simulink model "sm_boom_lift_crawler_harness_ground_manifold_hydr_debug"  (R2024b)
settings: Solver=ode23t  StartTime=0.0  StopTime=tVec.StopTime  FixedStep=2e-3  MaxStep=2  RelTol=1e-3  AbsTol=1e-3
PostLoadFcn:
  | sm_boom_lift_crawler_settest('chassis test')
StartFcn:
  | tic;
StopFcn:
  | Elapsed_Sim_Time = toc;
  | %disp(['Elapsed Sim Time = ' num2str(Elapsed_Sim_Time)]);
undefined symbols (not defined in the file): BasketR, Boom, Chassis, Extend, Jib, LevelM, LevelS, Lift, OutFL, OutFR, OutRL, OutRR, oVec, Tilt, TrackL, TrackR, Turret, tVec
libraries: sm_boom_lift_crawler_lib x22, fl_lib x15, sh_lib x15, nesl_utility x5, sm_lib x2, sm_boom_lift_crawler_lib_lift x1, sm_boom_lift_crawler_lib_inputs x1
(part 1 of 2)
Description:
  | Boom Lift Crawler Chassis with Hydraulic Actuation (Test Harness)
  | 
  | Copyright 2020-2024 The MathWorks, Inc.
settings Model: LastModifiedBy=smiller
settings SolverCC: AutoScaleAbsTol=off  AlgebraicLoopSolver=TrustRegion
settings DataIOCC: SignalLoggingName=logsout_sm_boom_lift_crawler
settings OptimizationCC: ReuseModelBlockBuffer=off
settings DebuggingCC: UnconnectedInputMsg=warning  UnconnectedOutputMsg=warning  UnconnectedLineMsg=warning
settings ModelReferenceCC: EnableRefExpFcnMdlSchedulingChecks=on
settings RTWCC: GPUComputeCapability=3.5  DLArmComputeVersion=19.05
settings SimscapeCC: SimscapeNominalValues="[{\"value\":\"1\",\"unit\":\"A\"},{\"value\":\"nomval_psi\",\"unit\":\"psi\"},{\"value\":\"1\",\"unit\":\"cm^2\"},{\"value\":\"nomval_cmv3_s\",\"unit\":\"cm^3/s\"},{\"value\":\"1\",\"unit\":\"kJ/kg\"},{\"value\":\"1\",\"unit\":\"kW\"},{\"value\":\"1\",\"unit\":\"l\"},{\"value\":\"nomval_N\",\"unit\":\"N\"},{\"value\":\"nomval_Nm\",\"unit\":\"N*m\"},{\"value\":\"1\",\"unit\":\"V\"}]"  SimscapeLogType=all  SimscapeLogName=simlog_sm_boom_lift_crawler  SimscapeLogLimitData=off  SimscapeOperatingPoint=op_hold4Sec_hydr
settings DiagnosticsConfigSet: SimMechanicsConflictingReferenceFrames=none  SimMechanicsRigidlyBoundBlock=none
settings ExplorerConfigSet: InternalSimMechanicsExplorerSettings="<ExplorerConfiguration><canonicalview>default</canonicalview><AnimationSetting><BasePlaybackSpeed>1.0</BasePlaybackSpeed><PlaybackSpeedFactor>8.0</PlaybackSpeedFactor></AnimationSetting><TilePanel><TileInfo><Tiles Columns=\"1\" Count=\"1\" Rows=\"1\"><Column Weight=\"1\"/><Row Weight=\"1\"/><Tile Height=\"1\" Width=\"1\" X=\"0\" Y=\"0\"/></Tiles></TileInfo><SceneInfo><SceneViewer><BGColor><R>1</R><G>1</G><B>1</B></BGColor><Camera><DoPerspective>on</DoPerspective><Position><X>-12.2424581714389937</X><Y>-0.143345264209557399</Y><Z>4.1505972342390427</Z></Position><Center><X>-4.62122899968606404</X><Y>-0.143345264209557399</Y><Z>4.15059723423904359</Z></Center><Up><X>0</X><Y>0</Y><Z>1</Z></Up><ViewLimDist>1</ViewLimDist><YLim>0.466307658154998583</YLim><XLim>0.828991392275552963</XLim></Camera></SceneViewer></SceneInfo></TilePanel><MechEditorPanel><Cameras><Camera><Id>Camera8</Id><Value><Name>Extend_Knuckle</Name><NativeCamera><PositionTrackingFeature>Lift.Boom.Arms.Telescope.Extend_Cylinder.Transform_Camera_Extend_Knuckle.F</PositionTrackingFeature><CenterTrackingFeature>Lift.Boom.Arms.Telescope.Extend_Cylinder.Transform_Camera_Extend_Knuckle.F</CenterTrackingFeature><UpVectorTrackingFeature>Lift.Boom.Arms.Telescope.Extend_Cylinder.Transform_Camera_Extend_Knuckle.F</UpVectorTrackingFeature><CenterTrackingOrigin>off</CenterTrackingOrigin><CenterTrackingDirection>-X</CenterTrackingDirection><UpVectorTrackingDirection>-Y</UpVectorTrackingDirection></NativeCamera></Value></Camera><Camera><Id>Camera9</Id><Value><Name>Extend_Basket</Name><NativeCamera><PositionTrackingFeature>Lift.Boom.Arms.Telescope.Extend_Cylinder.Transform_Camera_Extend_Basket.F</PositionTrackingFeature><CenterTrackingFeature>Lift.Boom.Arms.Telescope.Extend_Cylinder.Transform_Camera_Extend_Basket.F</CenterTrackingFeature><UpVectorTrackingFeature>Lift.Boom.Arms.Telescope.Extend_Cylinder.Transform_Camera_Extend_Basket.F</UpVectorTrackingFeature><CenterTrackingOrigin>off</CenterTrackingOrigin><CenterTrackingDirection>+X</CenterTrackingDirection><UpVectorTrackingDirection>+Y</UpVectorTrackingDirection></NativeCamera></Value></Camera><Camera><Id>Camera10</Id><Value><Name>Basket_Rotate</Name><NativeCamera><PositionTrackingFeature>Lift.Boom.Basket.Basket_Rotate.Bracket.Reference_Camera_Basket_Rotate_L.R</PositionTrackingFeature><CenterTrackingFeature>Lift.Boom.Basket.Basket_Rotate.Bracket.Reference_Camera_Basket_Rotate_L.R</CenterTrackingFeature><UpVectorTrackingFeature>Mech_Config.World.W</UpVectorTrackingFeature><CenterTrackingOrigin>off</CenterTrackingOrigin><CenterTrackingDirection>-X</CenterTrackingDirection><UpVectorTrackingDirection>+Z</UpVectorTrackingDirection></NativeCamera></Value></Camera><Camera><Id>Camera11</Id><Value><Name>Tilt_Knuckle</Name><NativeCamera><PositionTrackingFeature>Lift.Boom.Arms.Tower.Upper_Knuckle.Reference_Knuckle_Cam.R</PositionTrackingFeature><CenterTrackingFeature>Lift.Boom.Arms.Tower.Upper_Knuckle.Reference_Knuckle_Cam.R</CenterTrackingFeature><UpVectorTrackingFeature>Mech_Config.World.W</UpVectorTrackingFeature><CenterTrackingOrigin>off</CenterTrackingOrigin><CenterTrackingDirection>+Z</CenterTrackingDirection><UpVectorTrackingDirection>+Z</UpVectorTrackingDirection></NativeCamera></Value></Camera><Camera><Id>Camera12</Id><Value><Name>Full Test</Name><NativeCamera><PositionKeyframeSet><Keyframe><Time>0</Time><Value><X>-12.242458171438994</X><Y>-0.1433452642095574</Y><Z>4.1505972342390427</Z></Value></Keyframe><Keyframe><Time>69.026826430124729</Time><Value><X>-14.974593328379619</X><Y>0.0056652615564253064</Y><Z>5.3389029552684786</Z></Value></Keyframe><Keyframe><Time>110.29539843687829</Time><Value><X>-21.00761369699504</X><Y>-0.0057417156870510078</Y><Z>8.0689402037867488</Z></Value></Keyframe><Keyframe><Time>140.70430157635164</Time><Value><X>-31.272784439198116</X><Y>-2.5583130214499052e-10</Y><Z>12.723321478963756</Z></Value></Keyframe><Keyframe><Time>181.77628976806102</Time><Value><X>-31.272784439198116</X><Y>-2.5583130214499052e-10</Y><Z>12.723321478963756</Z></Value></Keyframe><Keyframe><Time>208.0087867386398</Time><Value><X>-23.351505250921551</X><Y>-2.5583182919801497e-10</Y><Z>9.1371534281977738</Z></Value></Keyframe><Keyframe><Time>243.06358572448306</Time><Value><X>-16.577121762622586</X><Y>-2.5583144573665537e-10</Y><Z>6.0702143126734844</Z></Value></Keyframe><Keyframe><Time>273.3415757110605</Time><Value><X>-16.577121762622586</X><Y>-2.5583144573665537e-10</Y><Z>6.0702143126734844</Z></Value></Keyframe><Keyframe><Time>321.2447002217541</Time><Value><X>-13.690590902490033</X><Y>0.01787769923724114</Y><Z>4.7891626503614262</Z></Value></Keyframe><Keyframe><Time>350</Time><Value><X>-13.690590902490033</X><Y>0.01787769923724114</Y><Z>4.7891626503614262</Z></Value></Keyframe></PositionKeyframeSet><CenterKeyframeSet><Keyframe><Time>0</Time><Value><X>-4.621228999686064</X><Y>-0.1433452642095574</Y><Z>4.1505972342390436</Z></Value></Keyframe><Keyframe><Time>69.026826430124729</Time><Value><X>-0.17395018713353672</X><Y>0.0056652615564253064</Y><Z>5.3389029552684786</Z></Value></Keyframe><Keyframe><Time>110.29539843687829</Time><Value><X>-9.0038066291239502</X><Y>-0.0057417156870549491</Y><Z>8.0689402037867524</Z></Value></Keyframe><Keyframe><Time>140.70430157635164</Time><Value><X>-14.136391845814327</X><Y>-2.5583979379462107e-10</Y><Z>12.72332147896376</Z></Value></Keyframe><Keyframe><Time>181.77628976806102</Time><Value><X>-2.3429975002054775</X><Y>-2.5584563781180217e-10</Y><Z>12.723321478963761</Z></Value></Keyframe><Keyframe><Time>208.0087867386398</Time><Value><X>-10.17575261115104</X><Y>-2.5583801743778167e-10</Y><Z>9.1371534281977755</Z></Value></Keyframe><Keyframe><Time>243.06358572448306</Time><Value><X>-0.54476849060194255</X><Y>-2.5583897563257738e-10</Y><Z>6.0702143126734844</Z></Value></Keyframe><Keyframe><Time>273.3415757110605</Time><Value><X>-0.11057247639663359</X><Y>-2.5583917956089291e-10</Y><Z>6.0702143126734844</Z></Value></Keyframe><Keyframe><Time>321.2447002217541</Time><Value><X>-5.3452949964231387</X><Y>0.017877699237237366</Y><Z>4.7891626503614253</Z></Value></Keyframe><Keyframe><Time>350</Time><Value><X>-5.3452949964231387</X><Y>0.017877699237237366</Y><Z>4.7891626503614253</Z></Value></Keyframe></CenterKeyframeSet><UpVectorKeyframeSet><Keyframe><Time>0</Time><Value><X>0</X><Y>0</Y><Z>1</Z></Value></Keyframe><Keyframe><Time>69.026826430124729</Time><Value><X>0</X><Y>0</Y><Z>1</Z></Value></Keyframe><Keyframe><Time>110.29539843687829</Time><Value><X>0</X><Y>0</Y><Z>1</Z></Value></Keyframe><Keyframe><Time>140.70430157635164</Time><Value><X>0</X><Y>0</Y><Z>1</Z></Value></Keyframe><Keyframe><Time>181.77628976806102</Time><Value><X>-2.0731981129868445e-16</X><Y>1.0273382740432149e-31</Y><Z>1</Z></Value></Keyframe><Keyframe><Time>208.0087867386398</Time><Value><X>1.4663775813922931e-57</X><Y>2.9591920320379324e-42</Y><Z>1</Z></Value></Keyframe><Keyframe><Time>243.06358572448306</Time><Value><X>1.3898401336634517e-57</X><Y>2.9591920320379324e-42</Y><Z>1</Z></Value></Keyframe><Keyframe><Time>273.3415757110605</Time><Value><X>1.3898401336605064e-57</X><Y>2.9591920320379324e-42</Y><Z>1</Z></Value></Keyframe><Keyframe><Time>321.2447002217541</Time><Value><X>1.3198478700492623e-57</X><Y>2.9591920320379324e-42</Y><Z>1</Z></Value></Keyframe><Keyframe><Time>350</Time><Value><X>1.0642863113510858e-16</X><Y>-4.813997747953607e-32</Y><Z>1</Z></Value></Keyframe></UpVectorKeyframeSet></NativeCamera></Value></Camera><Camera><Id>Camera13</Id><Value><Name>View_Basket_World</Name><NativeCamera><PositionTrackingFeature>Lift.Boom.Basket.Basket.Reference_Basket_Cam.R</PositionTrackingFeature><CenterTrackingFeature>Mech_Config.World.W</CenterTrackingFeature><UpVectorTrackingFeature>Lift.Boom.Basket.Basket.Reference_Basket_Cam.R</UpVectorTrackingFeature><CenterTrackingOrigin>on</CenterTrackingOrigin><UpVectorTrackingDirection>+Y</UpVectorTrackingDirection></NativeCamera></Value></Camera><Camera><Id>Camera14</Id><Value><Name>View_Worm_Drive</Name><NativeCamera><PositionTrackingFeature>Lift.Boom.Turret.Case.Reference_Worm_Cam.R</PositionTrackingFeature><CenterTrackingFeature>Lift.Boom.Turret.Case.Transform_Worm_Cam.B</CenterTrackingFeature><UpVectorTrackingFeature>Mech_Config.World.W</UpVectorTrackingFeature><CenterTrackingOrigin>on</CenterTrackingOrigin><UpVectorTrackingDirection>+Z</UpVectorTrackingDirection></NativeCamera></Value></Camera><Camera><Id>Camera15</Id><Value><Name>Extend_Retract_Pulley</Name><NativeCamera><PositionTrackingFeature>Lift.Boom.Arms.Telescope.Extend_Cylinder.Reference_Camera_Retract_Pulley.R</PositionTrackingFeature><CenterTrackingFeature>Lift.Boom.Arms.Telescope.Extend_Cylinder.Reference_Camera_Retract_Pulley.R</CenterTrackingFeature><UpVectorTrackingFeature>Lift.Boom.Arms.Telescope.Extend_Cylinder.Reference_Camera_Retract_Pulley.R</UpVectorTrackingFeature><CenterTrackingOrigin>off</CenterTrackingOrigin><CenterTrackingDirection>+Y</CenterTrackingDirection><UpVectorTrackingDirection>+Z</UpVectorTrackingDirection></NativeCamera></Value></Camera><Camera><Id>Camera16</Id><Value><Name>Extend_Extend_Pulley</Name><NativeCamera><PositionTrackingFeature>Lift.Boom.Arms.Telescope.Extend_Cylinder.Reference_Camera_Extend_Pulley.R</PositionTrackingFeature><CenterTrackingFeature>Lift.Boom.Arms.Telescope.Extend_Cylinder.Reference_Camera_Extend_Pulley.R</CenterTrackingFeature><UpVectorTrackingFeature>Lift.Boom.Arms.Telescope.Extend_Cylinder.Reference_Camera_Extend_Pulley.R</UpVectorTrackingFeature><CenterTrackingOrigin>off</CenterTrackingOrigin><CenterTrackingDirection>+Z</CenterTrackingDirection><UpVectorTrackingDirection>-Y</UpVectorTrackingDirection></NativeCamera></Value></Camera><Camera><Id>Camera17</Id><Value><Name>Jib</Name><NativeCamera><PositionTrackingFeature>Lift.Boom.Basket.Jib.Jib_Mount.Reference_Camera_Basket_Jib.R</PositionTrackingFeature><CenterTrackingFeature>Lift.Boom.Basket.Jib.Jib_Mount.Reference_Camera_Basket_Jib.R</CenterTrackingFeature><UpVectorTrackingFeature>Mech_Config.World.W</UpVectorTrackingFeature><CenterTrackingOrigin>off</CenterTrackingOrigin><CenterTrackingDirection>-X</CenterTrackingDirection><UpVectorTrackingDirection>+Z</UpVectorTrackingDirection></NativeCamera></Value></Camera></Cameras><GfxPanelCameraMap><MapElement CameraMLId=\"Camera12\" GfxPanelIndex=\"0\"/></GfxPanelCameraMap><VideoCreator><PlaybackSpeedRatio>8</PlaybackSpeedRatio><FrameRate>30</FrameRate><VideoFormat>MPEG-4</VideoFormat><FrameSize>auto</FrameSize></VideoCreator></MechEditorPanel></ExplorerConfiguration>"

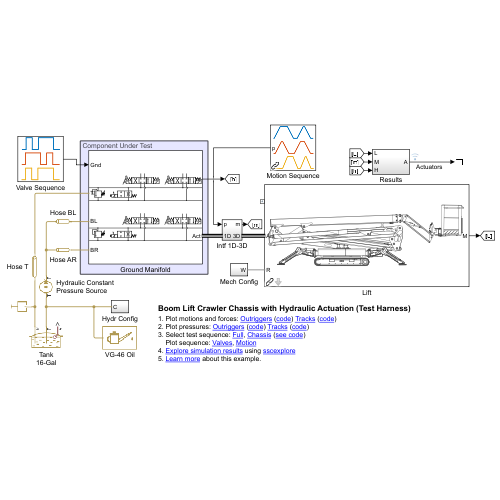
[thumbnail: Simulink's stored preview of the top-level diagram]
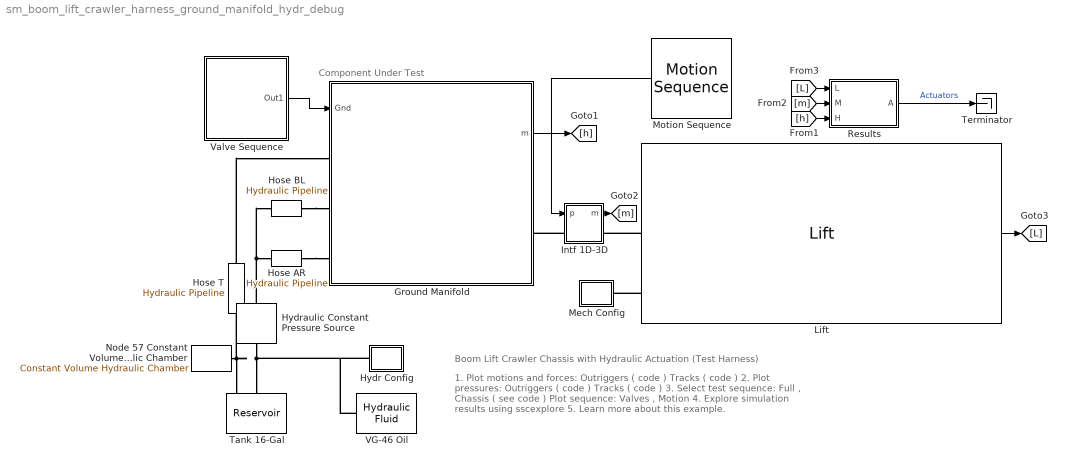
== system sm_boom_lift_crawler_harness_ground_manifold_hydr_debug ==
  note: Component Under Test
  note: Boom Lift Crawler Chassis with Hydraulic Actuation (Test Harness)
  note: 1. Plot motions and forces: Outriggers ( code ) Tracks ( code )
      | 2. Plot pressures: Outriggers ( code ) Tracks ( code )
      | 3. Select test sequence: Full , Chassis ( see code )
      | Plot sequence: Valves , Motion
      | 4. Explore simulation results using sscexplore
      | 5. Learn more about this example.
  Ground Manifold : Subsystem
      mask Display: image('sh004.svg')
  Hose AR : sh_lib/Pipelines/Hydraulic Pipeline  cs_type=1  d_in=lines.ground.main.d.p in  area=1e-4 m^2  D_h=1.12e-2 m  s_factor=64  length=lines.ground.main.l ft  length_ad=lines.ground.main.lr ft  roughness=15e-6 m  Re_lam=2000  Re_turb=4000  wall_type=1  pr_r_coef=2e-12 m/Pa  time_const=0.01 s  k_sh=1.4  initial_pressure=lines.ground.main.p0 psi
      settings: InternalSimscapePortConfiguration="{\"Bottom\":[],\"Left\":[{\"id\":\"A\",\"label\":\"A\",\"type\":\"foundation.hydraulic.hydraulic\"}],\"Right\":[{\"id\":\"B\",\"label\":\"B\",\"type\":\"foundation.hydraulic.hydraulic\"}],\"Top\":[]}"
  Hose BL : sh_lib/Pipelines/Hydraulic Pipeline  cs_type=1  d_in=lines.ground.main.d.p in  area=1e-4 m^2  D_h=1.12e-2 m  s_factor=64  length=lines.ground.main.l ft  length_ad=lines.ground.main.lr ft  roughness=15e-6 m  Re_lam=2000  Re_turb=4000  wall_type=1  pr_r_coef=2e-12 m/Pa  time_const=0.01 s  k_sh=1.4  initial_pressure=lines.ground.main.p0 psi
      settings: InternalSimscapePortConfiguration="{\"Bottom\":[],\"Left\":[{\"id\":\"A\",\"label\":\"A\",\"type\":\"foundation.hydraulic.hydraulic\"}],\"Right\":[{\"id\":\"B\",\"label\":\"B\",\"type\":\"foundation.hydraulic.hydraulic\"}],\"Top\":[]}"
  Hose T : sh_lib/Pipelines/Hydraulic Pipeline  cs_type=1  d_in=lines.ground.main.d.t in  area=1e-4 m^2  D_h=1.12e-2 m  s_factor=64  length=lines.ground.main.l ft  length_ad=lines.ground.main.lr ft  roughness=15e-6 m  Re_lam=2000  Re_turb=4000  wall_type=1  pr_r_coef=2e-12 m/Pa  time_const=0.01 s  k_sh=1.4  initial_pressure=lines.ground.main.p0 psi
      settings: InternalSimscapePortConfiguration="{\"Bottom\":[],\"Left\":[{\"id\":\"A\",\"label\":\"A\",\"type\":\"foundation.hydraulic.hydraulic\"}],\"Right\":[{\"id\":\"B\",\"label\":\"B\",\"type\":\"foundation.hydraulic.hydraulic\"}],\"Top\":[]}"
  Hydr Config : Subsystem
  Hydraulic Constant Pressure Source : fl_lib/Hydraulic/Hydraulic Sources/Hydraulic Constant Pressure Source  commanded_pressure=2e7 Pa
      settings: InternalSimscapePortConfiguration="{\"Bottom\":[],\"Left\":[{\"id\":\"P\",\"label\":\"P\",\"type\":\"foundation.hydraulic.hydraulic\"}],\"Right\":[{\"id\":\"T\",\"label\":\"T\",\"type\":\"foundation.hydraulic.hydraulic\"}],\"Top\":[]}"
  Intf 1D-3D : Subsystem
  Lift : sm_boom_lift_crawler_lib_lift/Lift  popup_gnd_outr=Force
  Mech Config : Subsystem
  Motion Sequence : sm_boom_lift_crawler_lib_inputs/Motion Sequence  SystemSampleTime=-1  VariantActivationTime=update diagram  AllowFlexibleInterface=on  Latency=0  AutoFrameSizeCalculation=off
  Node 57 Constant Volume Hydraulic Chamber : fl_lib/Hydraulic/Hydraulic Elements/Constant Volume Hydraulic Chamber  ch_sp=1  wall_type=1  ch_volume=1e-4 m^3  d_in=1e-2 m  length=1 m  pr_r_coef=1.2e-12 m/Pa  time_const=0.01 s  k_sh=1.4  pressure_specify=off  pressure_priority=High  pressure=0 Pa  pressure_nominal_specify=off  pressure_nominal_value=1  pressure_nominal_unit=Pa  diameter_incr_specify=off  diameter_incr_priority=High  diameter_incr=0 m  diameter_incr_nominal_specify=off  diameter_incr_nominal_value=1  diameter_incr_nominal_unit=m  flow_rate_specify=off  flow_rate_priority=None  flow_rate=0.001 m^3/s  flow_rate_nominal_specify=off  flow_rate_nominal_value=1  flow_rate_nominal_unit=m^3/s
      settings: InternalSimscapePortConfiguration="{\"Bottom\":[],\"Left\":[{\"id\":\"A\",\"label\":\"\",\"type\":\"foundation.hydraulic.hydraulic\"}],\"Right\":[],\"Top\":[]}"
  Results : Subsystem
  "Tank 16-Gal " : sh_lib/Hydraulic Utilities/Reservoir  press=0 psi  init_volume=16 gal  ret_diam=lines.ground.main.d.t in  loss_coeff=1
      settings: InternalSimscapePortConfiguration="{\"Bottom\":[],\"Left\":[{\"id\":\"V\",\"label\":\"V\",\"type\":\"output\"},{\"id\":\"P\",\"label\":\"P\",\"type\":\"foundation.hydraulic.hydraulic\"},{\"id\":\"R\",\"label\":\"R\",\"type\":\"foundation.hydraulic.hydraulic\"}],\"Right\":[],\"Top\":[]}"
  Terminator : Terminator
  VG-46 Oil : sh_lib/Hydraulic Utilities/Hydraulic Fluid  SelFluid=16  SysTemp=40  TrapAir=ratio_dissolved_air  ViscDerFactor=1  range_error=2
  Valve Sequence : Subsystem
      mask Display: image('sm_boom_lift_crawler_valve_seq_outputonly.svg');
  wires:
  Ground Manifold/1(m) -> [h]
  Results/1(A) -> Terminator/1  "Actuators"
  Lift/1 -> [L]
  Valve Sequence/1(Out1) -> Ground Manifold/1(Gnd)
  Motion Sequence/1 -> Intf 1D-3D/1(p)
  [h] -> Results/3(H)
  Intf 1D-3D/1(m) -> [m]
  [m] -> Results/2(M)
  [L] -> Results/1(L)
  connections:
  Hydraulic Constant Pressure Source/RConn1 -- "Tank 16-Gal "/LConn2 -- VG-46 Oil/RConn1 -- Hydr Config/RConn1
  Hose BL/RConn1 -- Ground Manifold/LConn2
  Intf 1D-3D/LConn1 -- Ground Manifold/RConn1
  Hose T/LConn1 -- Ground Manifold/LConn1
  Node 57 Constant Volume Hydraulic Chamber/LConn1 -- "Tank 16-Gal "/LConn3 -- Hose T/RConn1
  Hose AR/RConn1 -- Ground Manifold/LConn3
  Hydraulic Constant Pressure Source/LConn1 -- Hose AR/LConn1 -- Hose BL/LConn1
  Lift/LConn2 -- Intf 1D-3D/RConn1
  Lift/LConn3 -- Mech Config/LConn1

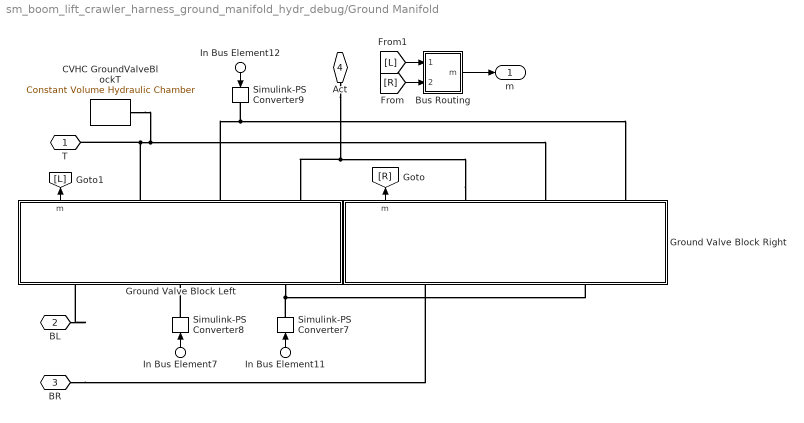
== system sm_boom_lift_crawler_harness_ground_manifold_hydr_debug/Ground Manifold ==
  In Bus Element7 : Inport  PortName=Gnd  Element=Tr
  In Bus Element11 : Inport  PortName=Gnd  Element=Ou
  In Bus Element12 : Inport  PortName=Gnd  Element=Pr
  Bus Routing : Subsystem
  CVHC GroundValveBlockT : fl_lib/Hydraulic/Hydraulic Elements/Constant Volume Hydraulic Chamber  ch_sp=1  wall_type=1  ch_volume=1e-4 m^3  d_in=1e-2 m  length=1 m  pr_r_coef=1.2e-12 m/Pa  time_const=0.01 s  k_sh=1.4  pressure_specify=off  pressure_priority=High  pressure=0 Pa  pressure_nominal_specify=off  pressure_nominal_value=1  pressure_nominal_unit=Pa  diameter_incr_specify=off  diameter_incr_priority=High  diameter_incr=0 m  diameter_incr_nominal_specify=off  diameter_incr_nominal_value=1  diameter_incr_nominal_unit=m  flow_rate_specify=off  flow_rate_priority=None  flow_rate=0.001 m^3/s  flow_rate_nominal_specify=off  flow_rate_nominal_value=1  flow_rate_nominal_unit=m^3/s
      settings: InternalSimscapePortConfiguration="{\"Bottom\":[],\"Left\":[{\"id\":\"A\",\"label\":\"\",\"type\":\"foundation.hydraulic.hydraulic\"}],\"Right\":[],\"Top\":[]}"
  Ground Valve Block Left : Subsystem
      mask Display: image('sh008.svg')
  Ground Valve Block Right : Subsystem
      mask Display: image('sh006.svg')
  Simulink-PS Converter7 : nesl_utility/Simulink-PS Converter  PhysicalDomain=network_engine_domain  SubClassName=ps_input  LeftPortType=input  RightPortType=output  PseudoPeriodic=off  Frequencies=[]  NoiseDistribution=none  NoiseParameters=[]  Unit=1  AffineConversion=off  FilteringAndDerivatives=provide  SimscapeFilterOrder=1  InputFilterTimeConstant=1  UdotUserProvided=0
  Simulink-PS Converter8 : nesl_utility/Simulink-PS Converter  PhysicalDomain=network_engine_domain  SubClassName=ps_input  LeftPortType=input  RightPortType=output  PseudoPeriodic=off  Frequencies=[]  NoiseDistribution=none  NoiseParameters=[]  Unit=1  AffineConversion=off  FilteringAndDerivatives=provide  SimscapeFilterOrder=1  InputFilterTimeConstant=1  UdotUserProvided=0
  Simulink-PS Converter9 : nesl_utility/Simulink-PS Converter  PhysicalDomain=network_engine_domain  SubClassName=ps_input  LeftPortType=input  RightPortType=output  PseudoPeriodic=off  Frequencies=[]  NoiseDistribution=none  NoiseParameters=[]  Unit=1  AffineConversion=off  FilteringAndDerivatives=provide  SimscapeFilterOrder=1  InputFilterTimeConstant=1  UdotUserProvided=0
  T : PMIOPort  Side=Left
  BL : PMIOPort  Port=2  Side=Left
  BR : PMIOPort  Port=3  Side=Left
  Act : PMIOPort  Port=4  Side=Right
  m : Outport
  wires:
  Ground Valve Block Right/1(m) -> [R]
  Ground Valve Block Left/1(m) -> [L]
  [L] -> Bus Routing/1(m1)
  [R] -> Bus Routing/2(m2)
  Bus Routing/1(m) -> m/1
  In Bus Element12/1 -> Simulink-PS Converter9/1
  In Bus Element11/1 -> Simulink-PS Converter7/1
  In Bus Element7/1 -> Simulink-PS Converter8/1
  connections:
  CVHC GroundValveBlockT/LConn1 -- Ground Valve Block Right/RConn2 -- T/RConn1 -- Ground Valve Block Left/RConn1
  BR/RConn1 -- Ground Valve Block Right/LConn1
  BL/RConn1 -- Ground Valve Block Left/LConn1
  Simulink-PS Converter9/RConn1 -- Ground Valve Block Right/RConn3 -- Ground Valve Block Left/RConn2
  Simulink-PS Converter7/RConn1 -- Ground Valve Block Right/LConn2 -- Ground Valve Block Left/LConn3
  Simulink-PS Converter8/RConn1 -- Ground Valve Block Left/LConn2
  Ground Valve Block Right/RConn1 -- Ground Valve Block Left/RConn3 -- Act/RConn1

== system sm_boom_lift_crawler_harness_ground_manifold_hydr_debug/Hydr Config ==
  Solver Configuration : nesl_utility/Solver Configuration  PhysicalDomain=network_engine_domain  SubClassName=solver  LeftPortType=input  RightPortType=generic  Tones=[]  Harmonics=[]  SimulateNoise=off  Profile=off  UseLocalSampling=off  EnableSwitchedLinearOptims=on  FrequencyDomain=off  UseCCode=off  RelTol=0.001  AbsTol=1e-06  MinStep=1e-09  ToWorkspace=off  RevertToSquareIcSolve=off  NumHomotopyIterations=100  PhasorMode=off  PhasorModeNumHarmonics=1  ConsistencySolver=NEWTON_FTOL  IndexReductionMethod=DerivativeReplacement  DoDC=off  ResidualTolerance=1e-9  ConsistencyTolSource=GLOBAL  ConsistencyAbsTol=0.001  ConsistencyRelTol=0.001  ConsistencyTolFactor=0.001  UseLocalSolver=off  LocalSolverChoice=NE_BACKWARD_EULER_ADVANCER  ResolveIndetEquations=on  FunctionEvalNumThread=1  LocalSolverSampleTime=2e-3  DoFixedCost=off  MaxNonlinIter=5  MaxModeIter=2  ComputeImpulses=off  ImpulseIterations=2  LinearAlgebra=Sparse  LinearAlgebraNumThread=0  EquationFormulation=NE_TIME_EF  DelaysMemoryBudget=1024  AutomaticFiltering=on  FilteringTimeConstant=1e-3  PartitionStorageMethod=EXHAUSTIVE  PartitionMemoryBudget=1024  PartitionMethod=FAST  MultibodyUseLocalSolver=off  MultibodyLocalSolverChoice=ODE1  MultibodyLocalSolverSampleTime=0.001
  C : PMIOPort  Side=Right
  connections:
  Solver Configuration/RConn1 -- C/RConn1

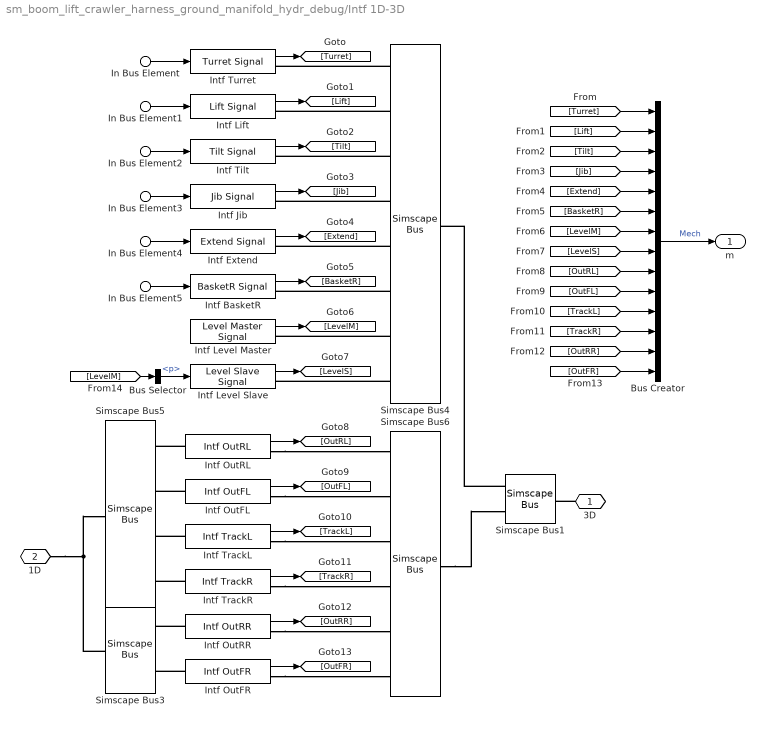
== system sm_boom_lift_crawler_harness_ground_manifold_hydr_debug/Intf 1D-3D ==
  In Bus Element : Inport  PortName=p  Element=Turret
  In Bus Element1 : Inport  PortName=p  Element=Lift
  In Bus Element2 : Inport  PortName=p  Element=Tilt
  In Bus Element3 : Inport  PortName=p  Element=Jib
  In Bus Element4 : Inport  PortName=p  Element=Extend
  In Bus Element5 : Inport  PortName=p  Element=BasketR
  Bus Creator : BusCreator  Inputs=14
  Bus Selector : BusSelector  OutputSignals=p
  Intf BasketR : sm_boom_lift_crawler_lib/BasketR Signal  SystemSampleTime=-1  VariantActivationTime=update diagram  AllowFlexibleInterface=on  Latency=0  AutoFrameSizeCalculation=off
  Intf Extend : sm_boom_lift_crawler_lib/Extend Signal  SystemSampleTime=-1  VariantActivationTime=update diagram  AllowFlexibleInterface=on  Latency=0  AutoFrameSizeCalculation=off
  Intf Jib : sm_boom_lift_crawler_lib/Jib Signal  SystemSampleTime=-1  VariantActivationTime=update diagram  AllowFlexibleInterface=on  Latency=0  AutoFrameSizeCalculation=off
  Intf Level Master : sm_boom_lift_crawler_lib/Level Master Signal  SystemSampleTime=-1  VariantActivationTime=update diagram  AllowFlexibleInterface=on  Latency=0  AutoFrameSizeCalculation=off
  Intf Level Slave : sm_boom_lift_crawler_lib/Level Slave Signal  SystemSampleTime=-1  VariantActivationTime=update diagram  AllowFlexibleInterface=on  Latency=0  AutoFrameSizeCalculation=off
  Intf Lift : sm_boom_lift_crawler_lib/Lift Signal  SystemSampleTime=-1  VariantActivationTime=update diagram  AllowFlexibleInterface=on  Latency=0  AutoFrameSizeCalculation=off
  Intf OutFL : sm_boom_lift_crawler_lib/Intf OutFL  SystemSampleTime=-1  VariantActivationTime=update diagram  AllowFlexibleInterface=on  Latency=0  AutoFrameSizeCalculation=off
  Intf OutFR : sm_boom_lift_crawler_lib/Intf OutFR  SystemSampleTime=-1  VariantActivationTime=update diagram  AllowFlexibleInterface=on  Latency=0  AutoFrameSizeCalculation=off
  Intf OutRL : sm_boom_lift_crawler_lib/Intf OutRL  SystemSampleTime=-1  VariantActivationTime=update diagram  AllowFlexibleInterface=on  Latency=0  AutoFrameSizeCalculation=off
  Intf OutRR : sm_boom_lift_crawler_lib/Intf OutRR  SystemSampleTime=-1  VariantActivationTime=update diagram  AllowFlexibleInterface=on  Latency=0  AutoFrameSizeCalculation=off
  Intf Tilt : sm_boom_lift_crawler_lib/Tilt Signal  SystemSampleTime=-1  VariantActivationTime=update diagram  AllowFlexibleInterface=on  Latency=0  AutoFrameSizeCalculation=off
  Intf TrackL : sm_boom_lift_crawler_lib/Intf TrackL  SystemSampleTime=-1  VariantActivationTime=update diagram  AllowFlexibleInterface=on  Latency=0  AutoFrameSizeCalculation=off
  Intf TrackR : sm_boom_lift_crawler_lib/Intf TrackR  SystemSampleTime=-1  VariantActivationTime=update diagram  AllowFlexibleInterface=on  Latency=0  AutoFrameSizeCalculation=off
  Intf Turret : sm_boom_lift_crawler_lib/Turret Signal  SystemSampleTime=-1  VariantActivationTime=update diagram  AllowFlexibleInterface=on  Latency=0  AutoFrameSizeCalculation=off
  Simscape Bus1 : SimscapeBus  HierarchyStrings=Boom;Chassis
  Simscape Bus3 : SimscapeBus  HierarchyStrings=OutRR;OutFR
  Simscape Bus4 : SimscapeBus  HierarchyStrings=Turret;Lift;Tilt;Jib;Extend;BasketR;LevelM;LevelS
  Simscape Bus5 : SimscapeBus  HierarchyStrings=OutRL;OutFL;TrackL;TrackR
  Simscape Bus6 : SimscapeBus  HierarchyStrings=OutRL;OutFL;TrackL;TrackR;OutRR;OutFR
  3D : PMIOPort  Side=Right
  1D : PMIOPort  Port=2  Side=Left
  m : Outport
  wires:
  [BasketR] -> Bus Creator/6
  [Jib] -> Bus Creator/4
  [LevelS] -> Bus Creator/8
  [TrackR] -> Bus Creator/12
  [Lift] -> Bus Creator/2
  [Tilt] -> Bus Creator/3
  [OutFL] -> Bus Creator/10
  [Turret] -> Bus Creator/1
  [LevelM] -> Bus Creator/7
  [TrackL] -> Bus Creator/11
  [OutRL] -> Bus Creator/9
  [Extend] -> Bus Creator/5
  [OutRR] -> Bus Creator/13
  [OutFR] -> Bus Creator/14
  Intf OutRL/1 -> [OutRL]
  Intf OutFL/1 -> [OutFL]
  Intf TrackL/1 -> [TrackL]
  Intf TrackR/1 -> [TrackR]
  Intf OutRR/1 -> [OutRR]
  Intf OutFR/1 -> [OutFR]
  Bus Creator/1 -> m/1  "Mech"
  In Bus Element5/1 -> Intf BasketR/1
  In Bus Element/1 -> Intf Turret/1
  Intf Turret/1 -> [Turret]
  [LevelM] -> Bus Selector/1
  In Bus Element4/1 -> Intf Extend/1
  Intf Level Master/1 -> [LevelM]
  In Bus Element3/1 -> Intf Jib/1
  Bus Selector/1 -> Intf Level Slave/1  "<p>"
  Intf Tilt/1 -> [Tilt]
  In Bus Element1/1 -> Intf Lift/1
  Intf Extend/1 -> [Extend]
  Intf BasketR/1 -> [BasketR]
  Intf Jib/1 -> [Jib]
  Intf Level Slave/1 -> [LevelS]
  Intf Lift/1 -> [Lift]
  In Bus Element2/1 -> Intf Tilt/1
  connections:
  3D/RConn1 -- Simscape Bus1/RConn1
  1D/RConn1 -- Simscape Bus3/RConn1 -- Simscape Bus5/RConn1
  Simscape Bus6/RConn1 -- Simscape Bus1/LConn2
  Intf OutFL/RConn1 -- Simscape Bus6/LConn2
  Intf OutFL/LConn1 -- Simscape Bus5/LConn2
  Intf OutRL/RConn1 -- Simscape Bus6/LConn1
  Intf OutRL/LConn1 -- Simscape Bus5/LConn1
  Intf TrackL/LConn1 -- Simscape Bus5/LConn3
  Intf TrackL/RConn1 -- Simscape Bus6/LConn3
  Intf TrackR/LConn1 -- Simscape Bus5/LConn4
  Intf TrackR/RConn1 -- Simscape Bus6/LConn4
  Intf OutFR/LConn1 -- Simscape Bus3/LConn2
  Intf OutFR/RConn1 -- Simscape Bus6/LConn6
  Intf OutRR/LConn1 -- Simscape Bus3/LConn1
  Intf OutRR/RConn1 -- Simscape Bus6/LConn5
  Simscape Bus1/LConn1 -- Simscape Bus4/RConn1
  Simscape Bus4/LConn6 -- Intf BasketR/RConn1
  Simscape Bus4/LConn3 -- Intf Tilt/RConn1
  Simscape Bus4/LConn2 -- Intf Lift/RConn1
  Simscape Bus4/LConn1 -- Intf Turret/RConn1
  Simscape Bus4/LConn5 -- Intf Extend/RConn1
  Simscape Bus4/LConn8 -- Intf Level Slave/RConn1
  Simscape Bus4/LConn7 -- Intf Level Master/RConn1
  Simscape Bus4/LConn4 -- Intf Jib/RConn1

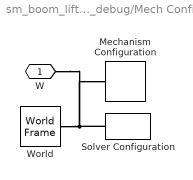
== system sm_boom_lift_crawler_harness_ground_manifold_hydr_debug/Mech Config ==
  Mechanism Configuration : sm_lib/Utilities/Mechanism Configuration  UniformGravity=Constant  GravityVector=[0 0 -9.80665]  GravityVectorUnits=m/s^2  LinearizationDelta=0.001  JointModeTransitionNonlinearIterations=2
  Solver Configuration : nesl_utility/Solver Configuration  PhysicalDomain=network_engine_domain  SubClassName=solver  LeftPortType=input  RightPortType=generic  Tones=[]  Harmonics=[]  SimulateNoise=off  Profile=off  UseLocalSampling=off  EnableSwitchedLinearOptims=on  FrequencyDomain=off  UseCCode=off  RelTol=0.001  AbsTol=1e-06  MinStep=1e-09  ToWorkspace=off  RevertToSquareIcSolve=off  NumHomotopyIterations=100  PhasorMode=off  PhasorModeNumHarmonics=1  ConsistencySolver=NEWTON_FTOL  IndexReductionMethod=DerivativeReplacement  DoDC=off  ResidualTolerance=1e-9  ConsistencyTolSource=GLOBAL  ConsistencyAbsTol=0.001  ConsistencyRelTol=0.001  ConsistencyTolFactor=0.001  UseLocalSolver=off  LocalSolverChoice=NE_BACKWARD_EULER_ADVANCER  ResolveIndetEquations=on  FunctionEvalNumThread=1  LocalSolverSampleTime=2e-3  DoFixedCost=off  MaxNonlinIter=3  MaxModeIter=2  ComputeImpulses=off  ImpulseIterations=2  LinearAlgebra=auto  LinearAlgebraNumThread=0  EquationFormulation=NE_TIME_EF  DelaysMemoryBudget=1024  AutomaticFiltering=on  FilteringTimeConstant=0.001  PartitionStorageMethod=AS_NEEDED  PartitionMemoryBudget=1024  PartitionMethod=ROBUST  MultibodyUseLocalSolver=off  MultibodyLocalSolverChoice=ODE1  MultibodyLocalSolverSampleTime=0.001
  World : sm_lib/Frames and Transforms/World Frame
  W : PMIOPort  Side=Left
  connections:
  Solver Configuration/RConn1 -- W/RConn1 -- Mechanism Configuration/RConn1 -- World/RConn1

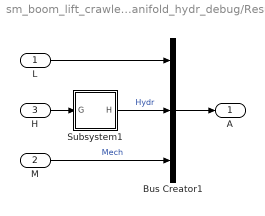
== system sm_boom_lift_crawler_harness_ground_manifold_hydr_debug/Results ==
  L : Inport
  M : Inport  Port=2
  H : Inport  Port=3
  Bus Creator1 : BusCreator  Inputs=3
  Subsystem1 : Subsystem
  A : Outport
  wires:
  Subsystem1/1(H) -> Bus Creator1/2  "Hydr"
  Bus Creator1/1 -> A/1
  H/1 -> Subsystem1/1(G)
  M/1 -> Bus Creator1/3  "Mech"
  L/1 -> Bus Creator1/1

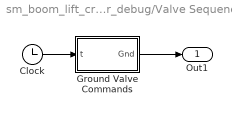
== system sm_boom_lift_crawler_harness_ground_manifold_hydr_debug/Valve Sequence ==
  Clock : Clock
  Ground Valve Commands : Subsystem
  Out1 : Outport
  wires:
  Clock/1 -> Ground Valve Commands/1(t)
  Ground Valve Commands/1(Gnd) -> Out1/1

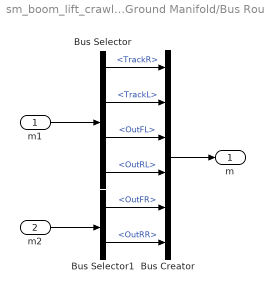
== system sm_boom_lift_crawler_harness_ground_manifold_hydr_debug/Ground Manifold/Bus Routing ==
  m1 : Inport
  m2 : Inport  Port=2
  Bus Creator : BusCreator  Inputs=6
  Bus Selector : BusSelector  OutputSignals=TrackR,TrackL,OutFL,OutRL
  Bus Selector1 : BusSelector  OutputSignals=OutFR,OutRR
  m : Outport
  wires:
  Bus Selector/4 -> Bus Creator/4  "<OutRL>"
  Bus Selector/3 -> Bus Creator/3  "<OutFL>"
  Bus Selector/2 -> Bus Creator/2  "<TrackL>"
  Bus Selector/1 -> Bus Creator/1  "<TrackR>"
  Bus Selector1/2 -> Bus Creator/6  "<OutRR>"
  Bus Selector1/1 -> Bus Creator/5  "<OutFR>"
  m2/1 -> Bus Selector1/1
  m1/1 -> Bus Selector/1
  Bus Creator/1 -> m/1

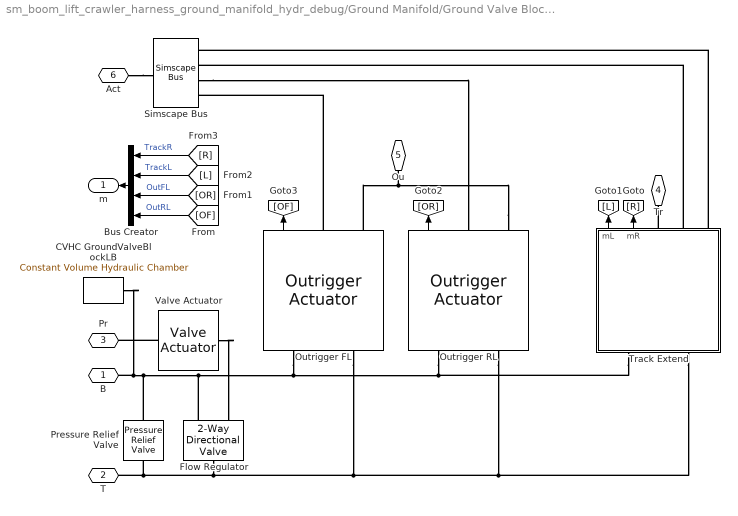
== system sm_boom_lift_crawler_harness_ground_manifold_hydr_debug/Ground Manifold/Ground Valve Block Left ==
  Bus Creator : BusCreator  Inputs=4
  CVHC GroundValveBlockLB : fl_lib/Hydraulic/Hydraulic Elements/Constant Volume Hydraulic Chamber  ch_sp=1  wall_type=1  ch_volume=1e-4 m^3  d_in=1e-2 m  length=1 m  pr_r_coef=1.2e-12 m/Pa  time_const=0.01 s  k_sh=1.4  pressure_specify=off  pressure_priority=High  pressure=0 Pa  pressure_nominal_specify=on  pressure_nominal_value=1  pressure_nominal_unit=Pa  diameter_incr_specify=off  diameter_incr_priority=High  diameter_incr=0 m  diameter_incr_nominal_specify=off  diameter_incr_nominal_value=1  diameter_incr_nominal_unit=m  flow_rate_specify=off  flow_rate_priority=None  flow_rate=0.001 m^3/s  flow_rate_nominal_specify=off  flow_rate_nominal_value=1  flow_rate_nominal_unit=m^3/s
      settings: InternalSimscapePortConfiguration="{\"Bottom\":[],\"Left\":[{\"id\":\"A\",\"label\":\"\",\"type\":\"foundation.hydraulic.hydraulic\"}],\"Right\":[],\"Top\":[]}"
  Flow Regulator : sh_lib/Valves/Directional Valves/2-Way Directional Valve  mdl_type=1  area_max=lines.ground.main.s.t in^2  opening_max=valves.control.l.max in  opening_tab=[-.002, 0, .002, .005, .015] m  area_tab=[1e-09, 2.0352e-07, 4.0736e-05, .00011438, .00034356] m^2  pressure_tab=[-10000000, -5000000, -2000000, 2000000, 5000000, 10000000] Pa  flow_rate_tab=[-1e-07, -7.0711e-08, -4.4721e-08, 4.4721e-08, 7.0711e-08, 1e-07; -2.0352e-05, -1.4391e-05, -9.1017e-06, 9.1017e-06, 1.4391e-05, 2.0352e-05; -.0040736, -.0028805, -.0018218, .0018218, .0028805, .0040736; -.011438, -.0080879, -.0051152, .0051152, .0080879, .011438; -.034356, -.024293, -.015364, .015364, .024293, .034356] m^3/s  interp_method=1  extrap_method=1  C_d=0.7  x_0=0 in  A_leak=1e-12 m^2  lam_spec=1  B_lam=0.999  Re_cr=12
      settings: InternalSimscapePortConfiguration="{\"Bottom\":[],\"Left\":[{\"id\":\"S\",\"label\":\"S\",\"type\":\"input\"},{\"id\":\"A\",\"label\":\"A\",\"type\":\"foundation.hydraulic.hydraulic\"}],\"Right\":[{\"id\":\"B\",\"label\":\"B\",\"type\":\"foundation.hydraulic.hydraulic\"}],\"Top\":[]}"
  Outrigger FL : sm_boom_lift_crawler_lib/Outrigger Actuator  SystemSampleTime=-1  VariantActivationTime=update diagram  AllowFlexibleInterface=on  Latency=0  AutoFrameSizeCalculation=off
  Outrigger RL : sm_boom_lift_crawler_lib/Outrigger Actuator  SystemSampleTime=-1  VariantActivationTime=update diagram  AllowFlexibleInterface=on  Latency=0  AutoFrameSizeCalculation=off
  Pressure Relief Valve : sh_lib/Valves/Pressure Control Valves/Pressure Relief Valve  valve_area_spec=1  p_diff_TLU=[30.15e5 : 15e3 : 31.35e5] Pa  area_TLU=[1 : 1 : 9] .* 1e-5 m^2  area_max=lines.ground.main.s.t in^2  pres_set=valves.relief.p.main psi  reg_range=valves.relief.dp psi  C_d=0.7  A_leak=1e-12 m^2  lam_spec=1  B_lam=0.999  Re_cr=12  dynamic=1  tau=0.1 s  area_init=1e-12 m^2
      settings: InternalSimscapePortConfiguration="{\"Bottom\":[],\"Left\":[{\"id\":\"A\",\"label\":\"A\",\"type\":\"foundation.hydraulic.hydraulic\"}],\"Right\":[{\"id\":\"B\",\"label\":\"B\",\"type\":\"foundation.hydraulic.hydraulic\"}],\"Top\":[]}"
  Simscape Bus : SimscapeBus  HierarchyStrings=TrackR;TrackL;OutRL;OutFL
  Track Extend : Subsystem
      mask Display: image('sh010.svg')
  Valve Actuator : sh_lib/Valves/Valve Actuators/Valve Actuator  valve_stroke=valves.control.l.max in  time_constant=valves.control.tau.c s  gain=1 in
      settings: InternalSimscapePortConfiguration="{\"Bottom\":[],\"Left\":[{\"id\":\"I\",\"label\":\"\",\"type\":\"input\"}],\"Right\":[{\"id\":\"O\",\"label\":\"\",\"type\":\"output\"}],\"Top\":[]}"
  B : PMIOPort  Side=Left
  T : PMIOPort  Port=2  Side=Right
  Pr : PMIOPort  Port=3  Side=Right
  Tr : PMIOPort  Port=4  Side=Left
  Ou : PMIOPort  Port=5  Side=Left
  Act : PMIOPort  Port=6  Side=Right
  m : Outport
  wires:
  Bus Creator/1 -> m/1
  [R] -> Bus Creator/1  "TrackR"
  [OF] -> Bus Creator/4  "OutRL"
  [OR] -> Bus Creator/3  "OutFL"
  [L] -> Bus Creator/2  "TrackL"
  Track Extend/2(mR) -> [R]
  Track Extend/1(mL) -> [L]
  Outrigger RL/1 -> [OR]
  Outrigger FL/1 -> [OF]
  connections:
  Valve Actuator/LConn1 -- Pr/RConn1
  Valve Actuator/RConn1 -- Flow Regulator/LConn1
  Outrigger RL/RConn2 -- Ou/RConn1 -- Outrigger FL/RConn2
  Track Extend/RConn1 -- Tr/RConn1
  Outrigger RL/LConn2 -- Track Extend/LConn2 -- Flow Regulator/RConn1 -- T/RConn1 -- Pressure Relief Valve/RConn1 -- Outrigger FL/LConn2
  Outrigger RL/LConn1 -- Track Extend/LConn1 -- Flow Regulator/LConn2 -- Pressure Relief Valve/LConn1 -- B/RConn1 -- CVHC GroundValveBlockLB/LConn1 -- Outrigger FL/LConn1
  Act/RConn1 -- Simscape Bus/RConn1
  Outrigger FL/RConn1 -- Simscape Bus/LConn4
  Simscape Bus/LConn3 -- Outrigger RL/RConn1
  Track Extend/RConn2 -- Simscape Bus/LConn2
  Track Extend/RConn3 -- Simscape Bus/LConn1

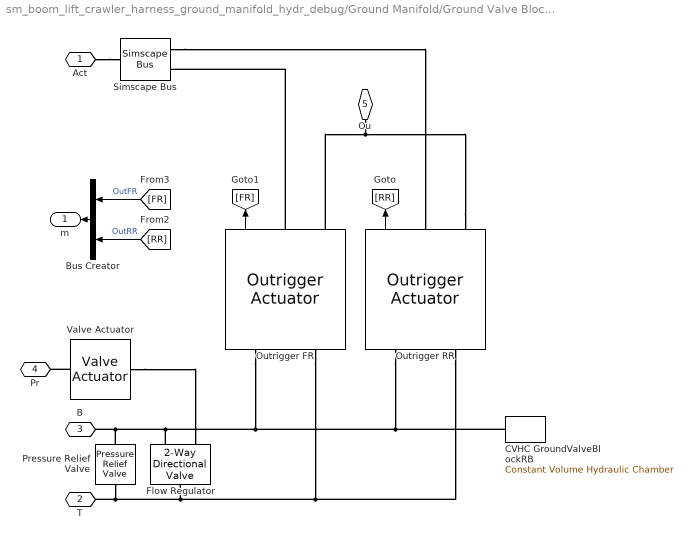
== system sm_boom_lift_crawler_harness_ground_manifold_hydr_debug/Ground Manifold/Ground Valve Block Right ==
  Bus Creator : BusCreator  Inputs=2
  "CVHC GroundValveBlockRB " : fl_lib/Hydraulic/Hydraulic Elements/Constant Volume Hydraulic Chamber  ch_sp=1  wall_type=1  ch_volume=1e-4 m^3  d_in=1e-2 m  length=1 m  pr_r_coef=1.2e-12 m/Pa  time_const=0.01 s  k_sh=1.4  pressure_specify=off  pressure_priority=High  pressure=0 Pa  pressure_nominal_specify=off  pressure_nominal_value=1  pressure_nominal_unit=Pa  diameter_incr_specify=off  diameter_incr_priority=High  diameter_incr=0 m  diameter_incr_nominal_specify=off  diameter_incr_nominal_value=1  diameter_incr_nominal_unit=m  flow_rate_specify=off  flow_rate_priority=None  flow_rate=0.001 m^3/s  flow_rate_nominal_specify=off  flow_rate_nominal_value=1  flow_rate_nominal_unit=m^3/s
      settings: InternalSimscapePortConfiguration="{\"Bottom\":[],\"Left\":[{\"id\":\"A\",\"label\":\"\",\"type\":\"foundation.hydraulic.hydraulic\"}],\"Right\":[],\"Top\":[]}"
  Flow Regulator : sh_lib/Valves/Directional Valves/2-Way Directional Valve  mdl_type=1  area_max=lines.ground.main.s.t in^2  opening_max=valves.control.l.max in  opening_tab=[-.002, 0, .002, .005, .015] m  area_tab=[1e-09, 2.0352e-07, 4.0736e-05, .00011438, .00034356] m^2  pressure_tab=[-10000000, -5000000, -2000000, 2000000, 5000000, 10000000] Pa  flow_rate_tab=[-1e-07, -7.0711e-08, -4.4721e-08, 4.4721e-08, 7.0711e-08, 1e-07; -2.0352e-05, -1.4391e-05, -9.1017e-06, 9.1017e-06, 1.4391e-05, 2.0352e-05; -.0040736, -.0028805, -.0018218, .0018218, .0028805, .0040736; -.011438, -.0080879, -.0051152, .0051152, .0080879, .011438; -.034356, -.024293, -.015364, .015364, .024293, .034356] m^3/s  interp_method=1  extrap_method=1  C_d=0.7  x_0=0 in  A_leak=1e-12 m^2  lam_spec=1  B_lam=0.999  Re_cr=12
      settings: InternalSimscapePortConfiguration="{\"Bottom\":[],\"Left\":[{\"id\":\"S\",\"label\":\"S\",\"type\":\"input\"},{\"id\":\"A\",\"label\":\"A\",\"type\":\"foundation.hydraulic.hydraulic\"}],\"Right\":[{\"id\":\"B\",\"label\":\"B\",\"type\":\"foundation.hydraulic.hydraulic\"}],\"Top\":[]}"
  Outrigger FR : sm_boom_lift_crawler_lib/Outrigger Actuator  SystemSampleTime=-1  VariantActivationTime=update diagram  AllowFlexibleInterface=on  Latency=0  AutoFrameSizeCalculation=off
  Outrigger RR : sm_boom_lift_crawler_lib/Outrigger Actuator  SystemSampleTime=-1  VariantActivationTime=update diagram  AllowFlexibleInterface=on  Latency=0  AutoFrameSizeCalculation=off
  Pressure Relief Valve : sh_lib/Valves/Pressure Control Valves/Pressure Relief Valve  valve_area_spec=1  p_diff_TLU=[30.15e5 : 15e3 : 31.35e5] Pa  area_TLU=[1 : 1 : 9] .* 1e-5 m^2  area_max=lines.ground.main.s.t in^2  pres_set=valves.relief.p.main psi  reg_range=valves.relief.dp psi  C_d=0.7  A_leak=1e-12 m^2  lam_spec=1  B_lam=0.999  Re_cr=12  dynamic=1  tau=0.1 s  area_init=1e-12 m^2
      settings: InternalSimscapePortConfiguration="{\"Bottom\":[],\"Left\":[{\"id\":\"A\",\"label\":\"A\",\"type\":\"foundation.hydraulic.hydraulic\"}],\"Right\":[{\"id\":\"B\",\"label\":\"B\",\"type\":\"foundation.hydraulic.hydraulic\"}],\"Top\":[]}"
  Simscape Bus : SimscapeBus  HierarchyStrings=OutRR;OutFR
  Valve Actuator : sh_lib/Valves/Valve Actuators/Valve Actuator  valve_stroke=valves.control.l.max in  time_constant=valves.control.tau.c s  gain=1 in
      settings: InternalSimscapePortConfiguration="{\"Bottom\":[],\"Left\":[{\"id\":\"I\",\"label\":\"\",\"type\":\"input\"}],\"Right\":[{\"id\":\"O\",\"label\":\"\",\"type\":\"output\"}],\"Top\":[]}"
  Act : PMIOPort  Side=Right
  T : PMIOPort  Port=2  Side=Right
  B : PMIOPort  Port=3  Side=Left
  Pr : PMIOPort  Port=4  Side=Right
  Ou : PMIOPort  Port=5  Side=Left
  m : Outport
  wires:
  Outrigger RR/1 -> [RR]
  Outrigger FR/1 -> [FR]
  [RR] -> Bus Creator/2  "OutRR"
  Bus Creator/1 -> m/1
  [FR] -> Bus Creator/1  "OutFR"
  connections:
  Valve Actuator/LConn1 -- Pr/RConn1
  Outrigger RR/RConn2 -- Ou/RConn1 -- Outrigger FR/RConn2
  Valve Actuator/RConn1 -- Flow Regulator/LConn1
  Flow Regulator/LConn2 -- Pressure Relief Valve/LConn1 -- B/RConn1 -- Outrigger RR/LConn1 -- "CVHC GroundValveBlockRB "/LConn1 -- Outrigger FR/LConn1
  Flow Regulator/RConn1 -- T/RConn1 -- Pressure Relief Valve/RConn1 -- Outrigger RR/LConn2 -- Outrigger FR/LConn2
  Act/RConn1 -- Simscape Bus/RConn1
  Outrigger FR/RConn1 -- Simscape Bus/LConn2
  Simscape Bus/LConn1 -- Outrigger RR/RConn1

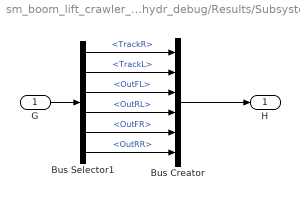
== system sm_boom_lift_crawler_harness_ground_manifold_hydr_debug/Results/Subsystem1 ==
  G : Inport
  Bus Creator : BusCreator  Inputs=6
  Bus Selector1 : BusSelector  OutputSignals=TrackR,TrackL,OutFL,OutRL,OutFR,OutRR
  H : Outport
  wires:
  Bus Creator/1 -> H/1
  G/1 -> Bus Selector1/1
  Bus Selector1/1 -> Bus Creator/1  "<TrackR>"
  Bus Selector1/2 -> Bus Creator/2  "<TrackL>"
  Bus Selector1/3 -> Bus Creator/3  "<OutFL>"
  Bus Selector1/4 -> Bus Creator/4  "<OutRL>"
  Bus Selector1/5 -> Bus Creator/5  "<OutFR>"
  Bus Selector1/6 -> Bus Creator/6  "<OutRR>"

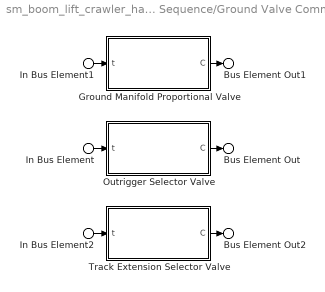
== system sm_boom_lift_crawler_harness_ground_manifold_hydr_debug/Valve Sequence/Ground Valve Commands ==
  In Bus Element : Inport  PortName=t
  In Bus Element1 : Inport  PortName=t
  In Bus Element2 : Inport  PortName=t
  Ground Manifold Proportional Valve : Subsystem
  Outrigger Selector Valve : Subsystem
  Track Extension Selector Valve : Subsystem
  Bus Element Out1 : Outport  VectorParamsAs1DForOutWhenUnconnected=off  PortName=Gnd  Element=Pr
  Bus Element Out : Outport  VectorParamsAs1DForOutWhenUnconnected=off  PortName=Gnd  Element=Ou
  Bus Element Out2 : Outport  VectorParamsAs1DForOutWhenUnconnected=off  PortName=Gnd  Element=Tr
  wires:
  In Bus Element/1 -> Outrigger Selector Valve/1(t)
  Track Extension Selector Valve/1(C) -> Bus Element Out2/1
  Ground Manifold Proportional Valve/1(C) -> Bus Element Out1/1
  In Bus Element2/1 -> Track Extension Selector Valve/1(t)
  In Bus Element1/1 -> Ground Manifold Proportional Valve/1(t)
  Outrigger Selector Valve/1(C) -> Bus Element Out/1
